simulink model "noplant"  (Simulink 7.9)
settings: Solver=ode45  StartTime=0.0  StopTime=10.0  RelTol=1e-3
undefined symbols (not defined in the file or in its folder): ARULE, LHS, PreNode, RHS, TransformationLib
libraries: Post_CommonlyUsedBlocks x7, Pre_CommonlyUsedBlocks x3
settings Model: Creator=jdenil  LastModifiedBy=jdenil

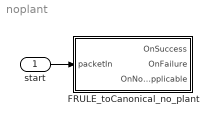
== system noplant ==
  start : Inport
  FRULE_toCanonical_no_plant : Subsystem  AncestorBlock=TransformationLib/ARULE
  wires:
  start/1 -> FRULE_toCanonical_no_plant/1(packetIn)

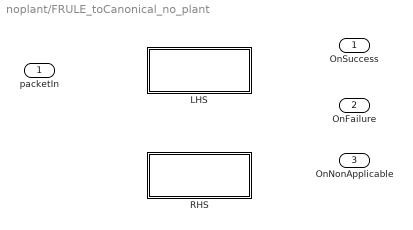
== system noplant/FRULE_toCanonical_no_plant ==
  packetIn : Inport
  LHS : Subsystem  AncestorBlock=TransformationLib/LHS  mask{Constraint=return True}
  RHS : Subsystem  AncestorBlock=TransformationLib/RHS  mask{Action=[]}
  OnSuccess : Outport
  OnFailure : Outport  Port=2
  OnNonApplicable : Outport  Port=3

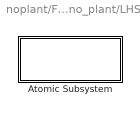
== system noplant/FRULE_toCanonical_no_plant/LHS ==
  Atomic Subsystem : Subsystem  AncestorBlock=Pre_CommonlyUsedBlocks/Atomic Subsystem  TreatAsAtomicUnit=on  mask{p_label=9, pre_Name=return False if 'plant' in attr_value else True}
      settings: AttributesFormatString=%<p_label>

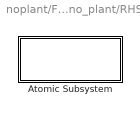
== system noplant/FRULE_toCanonical_no_plant/RHS ==
  Atomic Subsystem : Subsystem  AncestorBlock=Post_CommonlyUsedBlocks/Atomic Subsystem  TreatAsAtomicUnit=on  mask{p_label=9, post_Name=return attr_value}
      settings: AttributesFormatString=%<p_label>

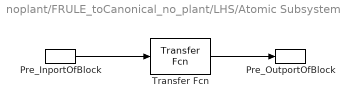
== system noplant/FRULE_toCanonical_no_plant/LHS/Atomic Subsystem ==
  Pre_InportOfBlock : Pre_CommonlyUsedBlocks/Pre_InportOfBlock  pre_label=1
      settings: AttributesFormatString=%<pre_label>
  Pre_OutportOfBlock : Pre_CommonlyUsedBlocks/Pre_OutportOfBlock  pre_label=3
      settings: AttributesFormatString=%<pre_label>
  Transfer Fcn : Pre_CommonlyUsedBlocks/Transfer Fcn  pre_label=2  pre_Name=return True  pre_Position=return True  pre_Numerator=return True  pre_Denominator=return True
      settings: AttributesFormatString=%<pre_label>
  wires:
  Pre_InportOfBlock/1 -> Transfer Fcn/1
  Transfer Fcn/1 -> Pre_OutportOfBlock/1

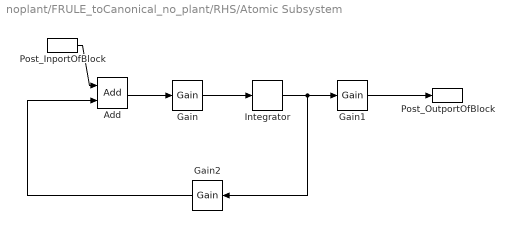
== system noplant/FRULE_toCanonical_no_plant/RHS/Atomic Subsystem ==
  Add : Post_CommonlyUsedBlocks/Add  post_label=4  post_Name=return PreNode('2')['Name']+'_add1'  post_Position=return PreNode('2')['Position']  post_Inputs=return '|++'
      settings: AttributesFormatString=%<post_label>
  Gain : Post_CommonlyUsedBlocks/Gain  post_label=5  post_gain=return PreNode('2')['Denominator'][0]  post_Name=return PreNode('2')['Name']+'_Gain_D2'  post_Position=return PreNode('2')['Position']
      settings: AttributesFormatString=%<post_label>
  Gain1 : Post_CommonlyUsedBlocks/Gain  post_label=7  post_gain=return PreNode('2')['Numerator'][0]  post_Name=return PreNode('2')['Name']+'Gain_N_1'  post_Position=return PreNode('2')['Position']
      settings: AttributesFormatString=%<post_label>
  Gain2 : Post_CommonlyUsedBlocks/Gain  post_label=8  post_gain=return -PreNode('2')['Denominator'][1]  post_Name=return PreNode('2')['Name']+'_Gain_D1'  post_Position=return PreNode('2')['Position']
      settings: AttributesFormatString=%<post_label>
  Integrator : Post_CommonlyUsedBlocks/Integrator  post_label=6  post_initial=return 0  post_Name=return PreNode('2')['Name']+'_int'  post_Position=return PreNode('2')['Position']
      settings: AttributesFormatString=%<post_label>
  Post_InportOfBlock : Post_CommonlyUsedBlocks/Post_InportOfBlock  post_label=1
      settings: AttributesFormatString=%<post_label>
  Post_OutportOfBlock : Post_CommonlyUsedBlocks/Post_OutportOfBlock  post_label=3
      settings: AttributesFormatString=%<post_label>
  wires:
  Post_InportOfBlock/1 -> Add/1
  Add/1 -> Gain/1
  Gain/1 -> Integrator/1
  Integrator/1 -> Gain2/1, Gain1/1
  Gain1/1 -> Post_OutportOfBlock/1
  Gain2/1 -> Add/2
